simulink model "BlockDiagram_Simple_Fluids_FirstPrinc"  (R2025b)
settings: Solver=VariableStepAuto  StartTime=0.0  StopTime=10.0  RelTol=1e-3
values from neighbouring files (symbols this model uses):
  P_amb = 101325    [init_engine_params.m]
  rho_f = 789    [init_engine_params.m]
  rho_ox = 988.82    [init_engine_params.m]
  V_c = 2.5335373958699e-4    (= 0.000253353739587)    [init_engine_params.m]
undefined symbols (not defined in the file or in its folder): CdA_max_f, P_feed_f, P_feed_ox
settings Model: Creator=gruby  LastModifiedBy=gruby

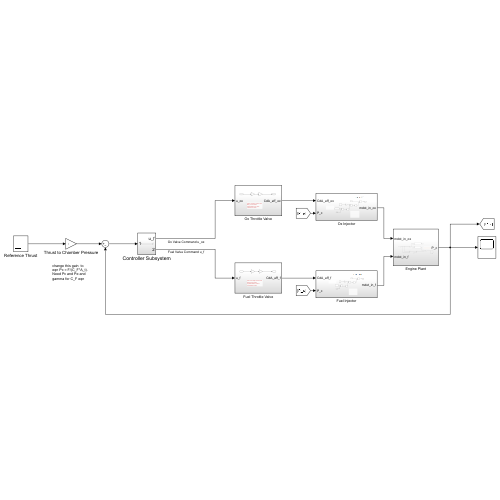
[thumbnail: Simulink's stored preview of the top-level diagram]
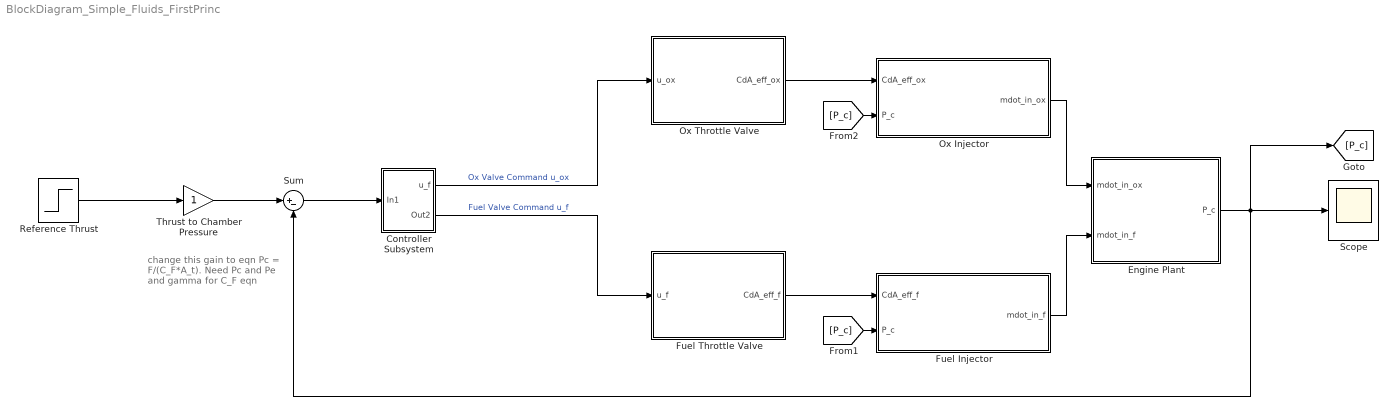
== system BlockDiagram_Simple_Fluids_FirstPrinc ==
  note: change this gain to eqn Pc = F/(C_F*A_t). Need Pc and Pe and gamma for C_F eqn
  Controller Subsystem : Subsystem
  Engine Plant : Subsystem
  Fuel Injector : Subsystem
  Fuel Throttle Valve : Subsystem
  Ox Injector : Subsystem
  Ox Throttle Valve : Subsystem
  Reference Thrust : Step  SampleTime=0
  Scope : Scope
      settings: ActiveDisplayYMinimum=-1.8374784378622904  ActiveDisplayYMaximum=16.537497604206919
  Sum : Sum  Inputs=|+-
  Thrust to Chamber Pressure : Gain
  wires:
  Sum/1 -> Controller Subsystem/1(In1)
  Thrust to Chamber Pressure/1 -> Sum/1
  Reference Thrust/1 -> Thrust to Chamber Pressure/1
  Engine Plant/1(P_c) -> Scope/1, [P_c], Sum/2
  [P_c] -> Fuel Injector/2(P_c)
  Controller Subsystem/1(u_f) -> Ox Throttle Valve/1(u_ox)  "Ox Valve Command u_ox"
  Controller Subsystem/2(Out2) -> Fuel Throttle Valve/1(u_f)  "Fuel Valve Command u_f"
  Fuel Throttle Valve/1(CdA_eff_f) -> Fuel Injector/1(CdA_eff_f)
  Ox Throttle Valve/1(CdA_eff_ox) -> Ox Injector/1(CdA_eff_ox)
  [P_c] -> Ox Injector/2(P_c)
  Fuel Injector/1(mdot_in_f) -> Engine Plant/2(mdot_in_f)
  Ox Injector/1(mdot_in_ox) -> Engine Plant/1(mdot_in_ox)

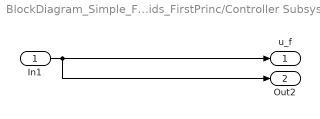
== system BlockDiagram_Simple_Fluids_FirstPrinc/Controller Subsystem ==
  In1 : Inport
  u_f : Outport
  Out2 : Outport  Port=2
  wires:
  In1/1 -> Out2/1, u_f/1

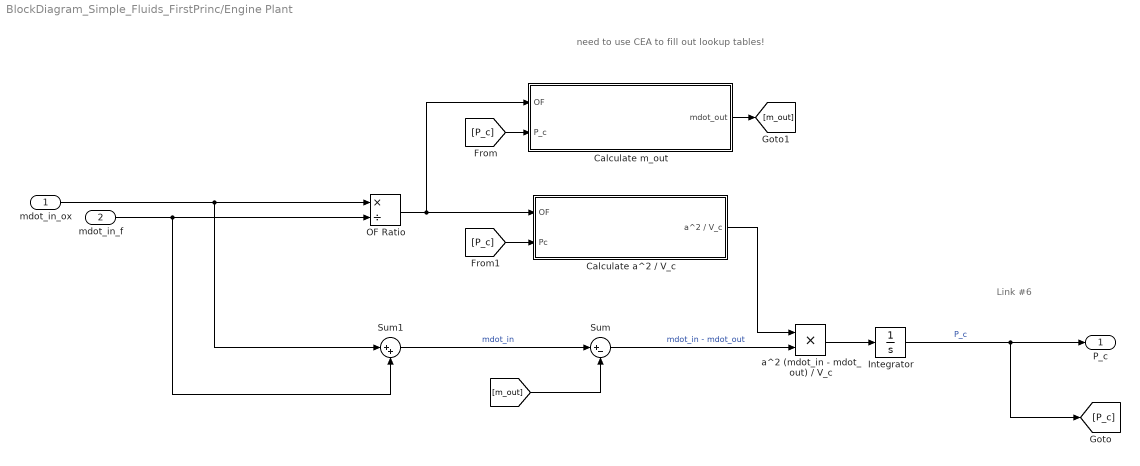
== system BlockDiagram_Simple_Fluids_FirstPrinc/Engine Plant ==
  note: Link #6
  note: need to use CEA to fill out lookup tables!
  mdot_in_ox : Inport
  mdot_in_f : Inport  Port=2
  Calculate a^2 / V_c : Subsystem
  Calculate m_out : Subsystem
  Integrator : Integrator  InitialCondition=P_amb
  OF Ratio : Product  Inputs=*/
  Sum : Sum  Inputs=|+-
  Sum1 : Sum  Inputs=|++
  "a^2 (mdot_in - mdot_out) / V_c " : Product
  P_c : Outport
  wires:
  mdot_in_f/1 -> Sum1/2, OF Ratio/2
  mdot_in_ox/1 -> Sum1/1, OF Ratio/1
  Sum/1 -> "a^2 (mdot_in - mdot_out) / V_c "/2  "mdot_in - mdot_out"
  Integrator/1 -> P_c/1, [P_c]  "P_c"
  OF Ratio/1 -> Calculate m_out/1(OF), Calculate a^2 / V_c/1(OF)
  Sum1/1 -> Sum/1  "mdot_in"
  "a^2 (mdot_in - mdot_out) / V_c "/1 -> Integrator/1
  [P_c] -> Calculate m_out/2(P_c)
  [P_c] -> Calculate a^2 / V_c/2(Pc)
  Calculate a^2 / V_c/1(a^2 / V_c) -> "a^2 (mdot_in - mdot_out) / V_c "/1
  Calculate m_out/1(mdot_out) -> [m_out]
  [m_out] -> Sum/2

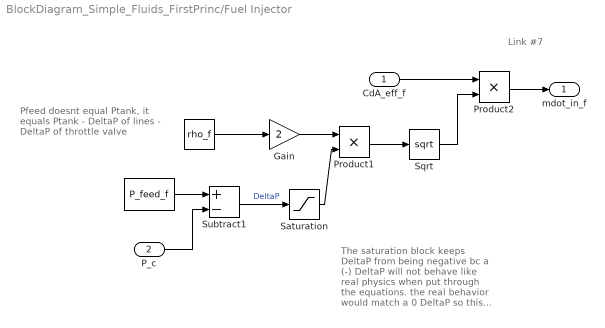
== system BlockDiagram_Simple_Fluids_FirstPrinc/Fuel Injector ==
  note: Link #7
  note: The saturation block keeps DeltaP from being negative bc a (-) DeltaP will not behave like real physics when put through the equations. the real behavior would match a 0 DeltaP so this makes a lower lim of 0.
  note: Pfeed doesnt equal Ptank, it equals Ptank - DeltaP of lines - DeltaP of throttle valve
  CdA_eff_f : Inport
  P_c : Inport  Port=2
  " " : Constant  Value=P_feed_f
  "  " : Constant  Value=rho_f
  Gain : Gain  Gain=2
  Product1 : Product
  Product2 : Product
  Saturation : Saturate  LowerLimit=0
  Sqrt : Sqrt
  Subtract1 : Sum  Inputs=+-
  mdot_in_f : Outport
  wires:
  Gain/1 -> Product1/1
  CdA_eff_f/1 -> Product2/1
  Subtract1/1 -> Saturation/1  "DeltaP"
  " "/1 -> Subtract1/1
  "  "/1 -> Gain/1
  Saturation/1 -> Product1/2
  Product1/1 -> Sqrt/1
  Sqrt/1 -> Product2/2
  P_c/1 -> Subtract1/2
  Product2/1 -> mdot_in_f/1

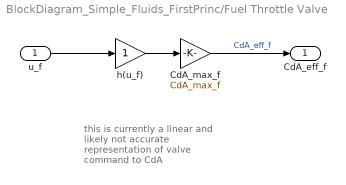
== system BlockDiagram_Simple_Fluids_FirstPrinc/Fuel Throttle Valve ==
  note: this is currently a linear and likely not accurate representation of valve command to CdA
  u_f : Inport
  CdA_max_f : Gain  Gain=CdA_max_f
  h(u_f) : Gain
  CdA_eff_f : Outport
  wires:
  h(u_f)/1 -> CdA_max_f/1
  CdA_max_f/1 -> CdA_eff_f/1  "CdA_eff_f"
  u_f/1 -> h(u_f)/1

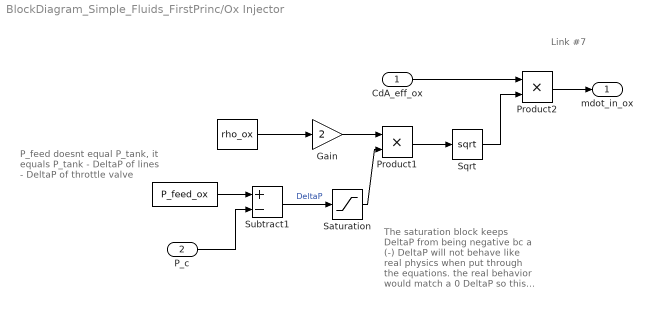
== system BlockDiagram_Simple_Fluids_FirstPrinc/Ox Injector ==
  note: Link #7
  note: The saturation block keeps DeltaP from being negative bc a (-) DeltaP will not behave like real physics when put through the equations. the real behavior would match a 0 DeltaP so this makes a lower lim of 0.
  note: P_feed doesnt equal P_tank, it equals P_tank - DeltaP of lines - DeltaP of throttle valve
  CdA_eff_ox : Inport
  P_c : Inport  Port=2
  " " : Constant  Value=P_feed_ox
  "  " : Constant  Value=rho_ox
  Gain : Gain  Gain=2
  Product1 : Product
  Product2 : Product
  Saturation : Saturate  LowerLimit=0
  Sqrt : Sqrt
  Subtract1 : Sum  Inputs=+-
  mdot_in_ox : Outport
  wires:
  Gain/1 -> Product1/1
  CdA_eff_ox/1 -> Product2/1
  Subtract1/1 -> Saturation/1  "DeltaP"
  " "/1 -> Subtract1/1
  "  "/1 -> Gain/1
  Saturation/1 -> Product1/2
  Product1/1 -> Sqrt/1
  Sqrt/1 -> Product2/2
  P_c/1 -> Subtract1/2
  Product2/1 -> mdot_in_ox/1

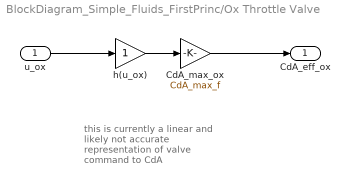
== system BlockDiagram_Simple_Fluids_FirstPrinc/Ox Throttle Valve ==
  note: this is currently a linear and likely not accurate representation of valve command to CdA
  u_ox : Inport
  CdA_max_ox : Gain  Gain=CdA_max_f
  h(u_ox) : Gain
  CdA_eff_ox : Outport
  wires:
  h(u_ox)/1 -> CdA_max_ox/1
  CdA_max_ox/1 -> CdA_eff_ox/1
  u_ox/1 -> h(u_ox)/1

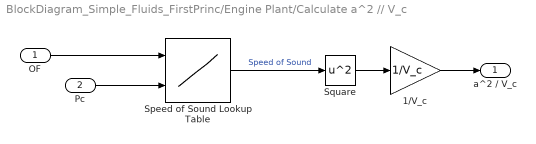
== system BlockDiagram_Simple_Fluids_FirstPrinc/Engine Plant/Calculate a^2 // V_c ==
  OF : Inport
  Pc : Inport  Port=2
  1/V_c : Gain  Gain=1/V_c
  Speed of Sound Lookup Table : Lookup_n-D  BreakpointsForDimension1=[1:3]  BreakpointsForDimension2=[1:3]  InternalRulePriority=Speed  RndMeth=Simplest
      settings: InputPortMap=u0,u1
  Square : Math  Operator=square
  a^2 / V_c : Outport
  wires:
  Speed of Sound Lookup Table/1 -> Square/1  "Speed of Sound"
  OF/1 -> Speed of Sound Lookup Table/1
  Square/1 -> 1/V_c/1
  Pc/1 -> Speed of Sound Lookup Table/2
  1/V_c/1 -> a^2 / V_c/1

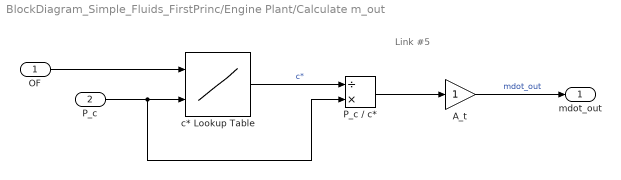
== system BlockDiagram_Simple_Fluids_FirstPrinc/Engine Plant/Calculate m_out ==
  note: Link #5
  OF : Inport
  P_c : Inport  Port=2
  A_t : Gain
  P_c / c* : Product  Inputs=/*
  c* Lookup Table : Lookup_n-D  BreakpointsForDimension1=[1:3]  BreakpointsForDimension2=[1:3]  InternalRulePriority=Speed  RndMeth=Simplest
      settings: InputPortMap=u0,u1
  mdot_out : Outport
  wires:
  c* Lookup Table/1 -> P_c / c*/1  "c*"
  P_c / c*/1 -> A_t/1
  OF/1 -> c* Lookup Table/1
  A_t/1 -> mdot_out/1  "mdot_out"
  P_c/1 -> P_c / c*/2, c* Lookup Table/2
